simulink model "Inverter_circuit_redesign_from_NITW_Paper23_compatible"  (R2021a)
settings: Solver=ode23t  StartTime=0.0  StopTime=2  RelTol=1e-3
values from neighbouring files (symbols this model uses):
  B = 5    [FOC_parameters_Basil.m]    (also in parameters_FOC.m = 53)
  C_LCL = 100e-6    (= 0.0001)    [FOC_parameters_Basil.m]
  D = 0.25    [FOC_parameters_Basil.m]    (also in parameters_FOC.m)
  k = 1    [FOC_parameters_Basil.m]
  L_LCL = 500e-6    (= 0.0005)    [FOC_parameters_Basil.m]
  Ll = 0.0416    [FOC_parameters_Basil.m]
  Lm = 0.0416    [FOC_parameters_Basil.m]    (also in parameters_FOC.m = 0.4)
  Lp = 0.0684    [FOC_parameters_Basil.m]
  M = 4.775    [FOC_parameters_Basil.m]    (also in parameters_FOC.m)
  P = 2    [FOC_parameters_Basil.m]    (also in parameters_FOC.m = 4)
  Rl = 0.976    [FOC_parameters_Basil.m]
  Rp = 1.298    [FOC_parameters_Basil.m]
  Tp = 0.027    [FOC_parameters_Basil.m]    (also in parameters_FOC.m = 0.0465)
  VDC = 800    [FOC_parameters_Basil.m]
undefined symbols (not defined in the file or in its folder): L
libraries: spsSeriesRLCBranchLib x9, pid_lib x6, spsIGBTDiodeLib x6, eeTransforms x4, spsCurrentMeasurementLib x3, simulink_extras x1, spsDCVoltageSourceLib x1, simulink x1, spsThreePhaseVIMeasurementLib x1, spsdq0toabcLib x1, spspowerguiLib x1
(part 1 of 2)
settings Model: SimulationMode=accelerator  Creator=Basilisk  LastModifiedBy=Basilisk

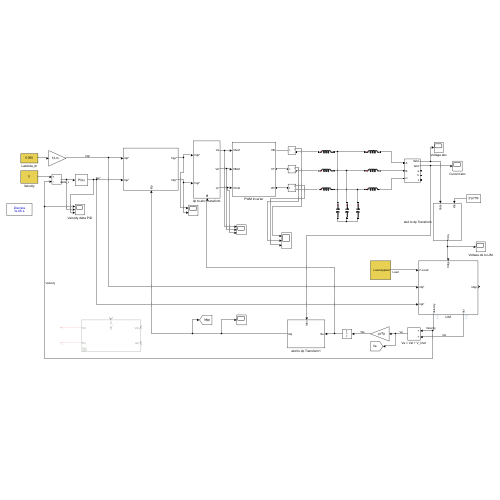
[thumbnail: Simulink's stored preview of the top-level diagram]
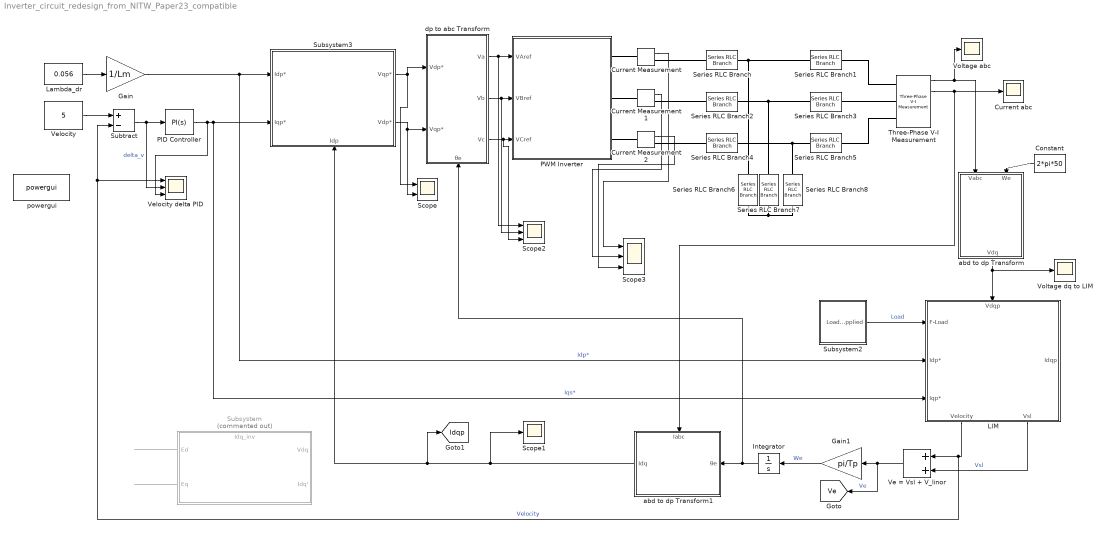
== system Inverter_circuit_redesign_from_NITW_Paper23_compatible ==
  Constant : Constant  Value=2*pi*50
  Current Measurement : spsCurrentMeasurementLib/Current Measurement  PhasorSimulation=off  OutputType=Complex  PSBequivalent=0
  Current Measurement1 : spsCurrentMeasurementLib/Current Measurement  PhasorSimulation=off  OutputType=Complex  PSBequivalent=0
  Current Measurement2 : spsCurrentMeasurementLib/Current Measurement  PhasorSimulation=off  OutputType=Complex  PSBequivalent=0
  Current abc : Scope
  Gain : Gain  Gain=1/Lm
  Gain1 : Gain  Gain=pi/Tp
  Integrator : Integrator
  LIM : Subsystem
      settings: PortSchema="{\"entries\":[{\"content\":{\"sides\":[{\"content\":{\"connectorIds\":[\"In1\",\"In2\",\"In3\"]},\"type\":\"ConnectorPlacement.EquallySpacedRectSide\",\"uuid\":\"f7446374-ee35-46fe-93ed-7921b6b2af41\"},{\"content\":{\"connectorIds\":[\"Out1\"],\"side\":\"RIGHT\"},\"type\":\"ConnectorPlacement.EquallySpacedRectSide\",\"uuid\":\"9c6022f9-7a1a-4d7e-a6a7-0d40c632aa44\"},{\"content\":{\"connectorIds\":[\"In4\"],\"side\":\"TOP\"},\"type\":\"ConnectorPlacement.EquallySpacedRectSide\",\"uuid\":\"61492046-b5c8-45e7-b8b1-17b26bfbb342\"},{\"content\":{\"connectorIds\":[\"Out2\",\"Out3\"],\"side\":\"BOTTOM\"},\"type\":\"ConnectorPlacement.EquallySpacedRectSide\",\"uuid\":\"5b9be1f1-04b7-4def-af6b-70d0d64eb3ec\"}]},\"type\":\"ConnectorPlacement.EquallySpacedConnector\",\"uuid\":\"408e196e-f76f-4ce9-bb6a-3d2dec3a79e2\"}],\"packageUris\":[\"http://schema.mathworks.com/mf0/Connector/R2020b\"],\"version\":\"1.0\"}"
  Lambda_dr : Constant  Value=0.056
  PID Controller : pid_lib/PID Controller  Controller=PI  Form=Parallel  TimeDomain=Continuous-time  UseExternalTs=off  SampleTime=-1  IntegratorMethod=Forward Euler  FilterMethod=Forward Euler  ControllerParametersSource=internal  P=10  I=5000  D=0  UseFilter=on  N=100  TunerSelectOption=Transfer Function Based (PID Tuner App)  InitialConditionSource=internal  InitialConditionForIntegrator=0  InitialConditionForFilter=0  DifferentiatorICPrevScaledInput=0  ExternalReset=none  TrackingMode=off  Kt=1  LimitOutput=off  SatLimitsSource=internal  UpperSaturationLimit=inf  LowerSaturationLimit=-inf  LinearizeAsGain=on  AntiWindupMode=none  Kb=1  POutMin=[]  POutMax=[]  IOutMin=[]  IOutMax=[]  DOutMin=[]  DOutMax=[]  NOutMin=[]  NOutMax=[]  SumOutMin=[]  SumOutMax=[]  SaturationOutMin=[]  SaturationOutMax=[]  PParamMin=[]  PParamMax=[]  IParamMin=[]  IParamMax=[]  DParamMin=[]  DParamMax=[]  NParamMin=[]  NParamMax=[]  KbParamMin=[]  KbParamMax=[]  KtParamMin=[]  KtParamMax=[]  KbOutMin=[]  KbOutMax=[]  KtOutMin=[]  KtOutMax=[]  IntegratorOutMin=[]  IntegratorOutMax=[]  FilterOutMin=[]  FilterOutMax=[]  SumI1OutMin=[]  SumI1OutMax=[]  SumI2OutMin=[]  SumI2OutMax=[]  SumI3OutMin=[]  SumI3OutMax=[]  SumI4OutMin=[]  SumI4OutMax=[]  SumDOutMin=[]  SumDOutMax=[]  DifferentiatorOutMin=[]  DifferentiatorOutMax=[]  FilterDiffOutCoefMin=[]  FilterDiffOutCoefMax=[]  ReciprocalOutMin=[]  ReciprocalOutMax=[]  SumDenOutMin=[]  SumDenOutMax=[]  SumNumOutMin=[]  SumNumOutMax=[]  DivideOutMin=[]  DivideOutMax=[]  UdiffTsProdOutMin=[]  UdiffTsProdOutMax=[]  NTsProdOutMin=[]  NTsProdOutMax=[]  UintegralTsProdOutMin=[]  UintegralTsProdOutMax=[]  UngainTsProdOutMin=[]  UngainTsProdOutMax=[]  IntegratorContinuousStateAttributes=''  IntegratorStateMustResolveToSignalObject=off  IntegratorRTWStateStorageClass=Auto  FilterContinuousStateAttributes=''  FilterStateMustResolveToSignalObject=off  FilterRTWStateStorageClass=Auto  ParallelPVariant=InternalParameters  IdealPVariant=Disabled  IVariant=InternalParameters  DVariant=Disabled  IntegratorVariant=Continuous  SatVariant=Disabled  AWVariant=Passthrough  PCopyVariant=Disabled  TRVariant=Disabled  FdbkBlocksVariant=Forward  IdealPFdbkVariant=Disabled  SatFdbkVariant=Disabled  DerivativeFilterVariant=Disabled  NVariant=Disabled  NCopyVariant=Disabled_SignalSpec  FilterICVariant=Disabled  IntegratorICVariant=InternalICs  ExternalResetVariant=Disabled  TRSumVariant=Passthrough  SumFdbkVariant=Disabled  SumVariant=Sum_PI  TsampFilterVariant=InternalTs  TsampNgainVariant=Passthrough  TsampIntegralVariant=Passthrough  ExternalSaturationOutDataTypeStr=Inherit: Same as second input
  PWM Inverter : Subsystem
  Scope : Scope  NumInputPorts=2
  Scope1 : Scope
  Scope2 : Scope  NumInputPorts=3
  Scope3 : Scope  NumInputPorts=3
  Series RLC Branch{,1..5} (6 alike) : spsSeriesRLCBranchLib/Series RLC Branch  LConnTagsString=__new0  RConnTagsString=__new0  BranchType=L  Resistance=1  Inductance=L_LCL  SetiL0=off  InitialCurrent=0  Capacitance=1e-6  Setx0=off  InitialVoltage=0  Measurements=None
  Series RLC Branch6 : spsSeriesRLCBranchLib/Series RLC Branch  LConnTagsString=__new0  RConnTagsString=__new0  BranchType=C  Resistance=1  Inductance=L  SetiL0=off  InitialCurrent=0  Capacitance=C_LCL  Setx0=off  InitialVoltage=0  Measurements=None
  Series RLC Branch7 : spsSeriesRLCBranchLib/Series RLC Branch  LConnTagsString=__new0  RConnTagsString=__new0  BranchType=C  Resistance=1  Inductance=L  SetiL0=off  InitialCurrent=0  Capacitance=C_LCL  Setx0=off  InitialVoltage=0  Measurements=None
  Series RLC Branch8 : spsSeriesRLCBranchLib/Series RLC Branch  LConnTagsString=__new0  RConnTagsString=__new0  BranchType=C  Resistance=1  Inductance=L  SetiL0=off  InitialCurrent=0  Capacitance=C_LCL  Setx0=off  InitialVoltage=0  Measurements=None
  Subsystem : Subsystem  Commented=on
      settings: PortSchema="{\"entries\":[{\"content\":{\"sides\":[{\"content\":{\"connectorIds\":[\"Out1\",\"Out2\"]},\"type\":\"ConnectorPlacement.EquallySpacedRectSide\",\"uuid\":\"49878900-a608-4033-9c06-f0f879ae24be\"},{\"content\":{\"connectorIds\":[\"In2\",\"In3\"],\"side\":\"RIGHT\"},\"type\":\"ConnectorPlacement.EquallySpacedRectSide\",\"uuid\":\"696fb92a-6e5e-4f05-bb0c-e09c99220dcc\"},{\"content\":{\"connectorIds\":[\"In1\"],\"side\":\"TOP\"},\"type\":\"ConnectorPlacement.EquallySpacedRectSide\",\"uuid\":\"dec37822-b677-40af-afbd-2d2c67f7ec3b\"}]},\"type\":\"ConnectorPlacement.EquallySpacedConnector\",\"uuid\":\"87482552-0ae1-4097-8c32-6cc01319ff44\"}],\"packageUris\":[\"http://schema.mathworks.com/mf0/Connector/R2020b\"],\"version\":\"1.0\"}"
  Subsystem2 : Subsystem
  Subsystem3 : Subsystem
      settings: PortSchema="{\"entries\":[{\"content\":{\"sides\":[{\"content\":{\"connectorIds\":[\"In1\",\"In2\"]},\"type\":\"ConnectorPlacement.EquallySpacedRectSide\",\"uuid\":\"297be966-0d57-4ba3-8372-2661d6cd0aff\"},{\"content\":{\"connectorIds\":[\"Out1\",\"Out2\"],\"side\":\"RIGHT\"},\"type\":\"ConnectorPlacement.EquallySpacedRectSide\",\"uuid\":\"6bb0515e-c942-4d41-9641-f6064e864ee1\"},{\"content\":{\"connectorIds\":[],\"side\":\"TOP\"},\"type\":\"ConnectorPlacement.EquallySpacedRectSide\",\"uuid\":\"b418268d-3115-4ff4-b82e-d56401585d58\"},{\"content\":{\"connectorIds\":[\"In3\"],\"side\":\"BOTTOM\"},\"type\":\"ConnectorPlacement.EquallySpacedRectSide\",\"uuid\":\"fdde8d49-e3fc-403e-acf2-e5bf672785bb\"}]},\"type\":\"ConnectorPlacement.EquallySpacedConnector\",\"uuid\":\"bea3ecdb-df2c-4728-adcd-4b82f3cb5d95\"}],\"packageUris\":[\"http://schema.mathworks.com/mf0/Connector/R2020b\"],\"version\":\"1.0\"}"
  Subtract : Sum  Inputs=+-
  Three-Phase V-I Measurement : spsThreePhaseVIMeasurementLib/Three-Phase V-I Measurement  VoltageMeasurement=phase-to-phase  SetLabelV=off  LabelV=Vabc  Vpu=off  VpuLL=off  CurrentMeasurement=yes  SetLabelI=off  LabelI=Iabc  Ipu=off  Pbase=100e6  Vbase=500e3  OutputType=Complex  PhasorSimulation=off  PSBequivalent=0
  Ve = Vsl + V_linor : Sum
  Velocity : Constant  Value=5
  Velocity delta PID : Scope  NumInputPorts=3
  Voltage abc : Scope
  Voltage dq to LIM : Scope
  abd to dp Transform : Subsystem
  abd to dp Transform1 : Subsystem
      settings: PortSchema="{\"entries\":[{\"content\":{\"sides\":[{\"content\":{\"connectorIds\":[\"Out1\"]},\"type\":\"ConnectorPlacement.EquallySpacedRectSide\",\"uuid\":\"0a5c08c4-5c41-497e-b18e-e04a9254d192\"},{\"content\":{\"connectorIds\":[\"In2\"],\"side\":\"RIGHT\"},\"type\":\"ConnectorPlacement.EquallySpacedRectSide\",\"uuid\":\"782de88f-5f2e-44b5-b7d6-55f2bd67aa91\"},{\"content\":{\"connectorIds\":[],\"side\":\"TOP\"},\"type\":\"ConnectorPlacement.EquallySpacedRectSide\",\"uuid\":\"cedc65d0-c52b-4972-ac1b-f9f495532484\"},{\"content\":{\"connectorIds\":[\"In1\"],\"side\":\"BOTTOM\"},\"type\":\"ConnectorPlacement.EquallySpacedRectSide\",\"uuid\":\"096e216c-1e33-4a9a-a102-8d40bb808988\"}]},\"type\":\"ConnectorPlacement.EquallySpacedConnector\",\"uuid\":\"2e2ddd2f-c989-4eb0-a4d7-2b4ecf545aeb\"}],\"packageUris\":[\"http://schema.mathworks.com/mf0/Connector/R2020b\"],\"version\":\"1.0\"}"
  dp to abc Transform : Subsystem
      settings: PortSchema="{\"entries\":[{\"content\":{\"sides\":[{\"content\":{\"connectorIds\":[\"In1\",\"In2\"]},\"type\":\"ConnectorPlacement.EquallySpacedRectSide\",\"uuid\":\"d8a782e4-9ec4-4209-9b4b-b1627326e2fd\"},{\"content\":{\"connectorIds\":[\"Out1\",\"Out2\",\"Out3\"],\"side\":\"RIGHT\"},\"type\":\"ConnectorPlacement.EquallySpacedRectSide\",\"uuid\":\"69fe3e47-1152-49e6-a7ef-958cf96a3504\"},{\"content\":{\"connectorIds\":[],\"side\":\"TOP\"},\"type\":\"ConnectorPlacement.EquallySpacedRectSide\",\"uuid\":\"f13122e8-6ec9-4b07-81b4-0ba679e15a5f\"},{\"content\":{\"connectorIds\":[\"In3\"],\"side\":\"BOTTOM\"},\"type\":\"ConnectorPlacement.EquallySpacedRectSide\",\"uuid\":\"3a3b978b-03f4-40da-8c91-f6bb64aea85e\"}]},\"type\":\"ConnectorPlacement.EquallySpacedConnector\",\"uuid\":\"570f73f2-39cb-4994-9999-9a17a3f46023\"}],\"packageUris\":[\"http://schema.mathworks.com/mf0/Connector/R2020b\"],\"version\":\"1.0\"}"
  powergui : spspowerguiLib/powergui  Priority=1  SimulationMode=Discrete  SampleTime=1e-6  frequency=60  Iterations=50  frequencyindice=0  Pbase=100e6  ErrMax=1e-4  UnitsV=kV  UnitsW=MW  buscounter=0  FunctionMessages=off  echomessages=off  EnableUseOfTLC=off  CurrentSourceSwitches=off  DisableSnubberDevices=off  DisableRonSwitches=off  DisableVfSwitches=off  DisplayEquations=off  AutomaticDiscreteSolvers=off  SolverType=Tustin/Backward Euler (TBE)  Interpol=off  ExternalGateDelay=off  methode=off  Ts=100  x0status=blocks  SPID=on  SwTol=0  HookPort=off  NonlinearTolerance=1e-4  nMaxIteration=100  ContinueOnMaxIteration=off  RestoreLinks=warning  ResistiveCurrentMeasurement=off  Frange=[0:2:500]  Ylog=off  Xlog=on  ShowGrid=off  save=off  variable=ZData  structure=0  ZoomFFT=off  StartTime=0.0  cycles=1  DisplayStyle=1  fundamental=60  FreqAxis=off  MaxFrequency=1000  frequencyindicesteady=1  RmsSteady=1  display=off
  tag scope: Idqp=global, Ve=global
  wires:
  abd to dp Transform/1(Vdq) -> Voltage dq to LIM/1, LIM/4(Vdqp)
  Constant/1 -> abd to dp Transform/1(We)
  Three-Phase V-I Measurement/1 -> Voltage abc/1, abd to dp Transform/2(Vabc)
  Subsystem/1(Ed) -> ?
  Subsystem/2(Eq) -> ?
  Velocity/1 -> Subtract/1
  Subsystem2/1(Load Applied) -> LIM/1(F-Load)  "Load"
  Integrator/1 -> abd to dp Transform1/2(θe), dp to abc Transform/3(θe)
  LIM/2(Velocity) -> Velocity delta PID/1, Subtract/2, Ve = Vsl + V_linor/1  "Velocity"
  LIM/3(Vsl) -> Ve = Vsl + V_linor/2  "Vsl"
  Subtract/1 -> PID Controller/1, Velocity delta PID/2  "delta_v"
  PID Controller/1 -> Velocity delta PID/3, LIM/3(Iqp*), Subsystem3/2(Iqp*)  "Iqs*"
  Lambda_dr/1 -> Gain/1
  Gain/1 -> LIM/2(Idp*), Subsystem3/1(Idp*)  "Idp*"
  Gain1/1 -> Integrator/1  "We"
  Ve = Vsl + V_linor/1 -> [Ve], Gain1/1  "Ve"
  Subsystem3/2(Vdp*) -> Scope/2, dp to abc Transform/2(Vqp*)
  Subsystem3/1(Vqp*) -> Scope/1, dp to abc Transform/1(Vdp*)
  dp to abc Transform/1(Va) -> Scope2/1, PWM Inverter/1(VAref)
  dp to abc Transform/2(Vb) -> Scope2/2, PWM Inverter/2(VBref)
  dp to abc Transform/3(Vc) -> Scope2/3, PWM Inverter/3(VCref)
  abd to dp Transform1/1(Idq) -> Scope1/1, [Idqp], Subsystem3/3(Idp)
  Three-Phase V-I Measurement/2 -> abd to dp Transform1/1(Iabc), Current abc/1
  Current Measurement/1 -> Scope3/1
  Current Measurement1/1 -> Scope3/2
  Current Measurement2/1 -> Scope3/3
  connections:
  Series RLC Branch/LConn1 -- Current Measurement/RConn1
  Series RLC Branch1/LConn1 -- Series RLC Branch6/LConn1 -- Series RLC Branch/RConn1
  Series RLC Branch2/LConn1 -- Current Measurement1/RConn1
  Series RLC Branch3/LConn1 -- Series RLC Branch2/RConn1 -- Series RLC Branch7/LConn1
  Series RLC Branch4/LConn1 -- Current Measurement2/RConn1
  Series RLC Branch5/LConn1 -- Series RLC Branch8/LConn1 -- Series RLC Branch4/RConn1
  Series RLC Branch6/RConn1 -- Series RLC Branch7/RConn1 -- Series RLC Branch8/RConn1
  Three-Phase V-I Measurement/LConn1 -- Series RLC Branch1/RConn1
  Three-Phase V-I Measurement/LConn2 -- Series RLC Branch3/RConn1
  Three-Phase V-I Measurement/LConn3 -- Series RLC Branch5/RConn1
  PWM Inverter/RConn1 -- Current Measurement/LConn1
  Current Measurement1/LConn1 -- PWM Inverter/RConn2
  PWM Inverter/RConn3 -- Current Measurement2/LConn1

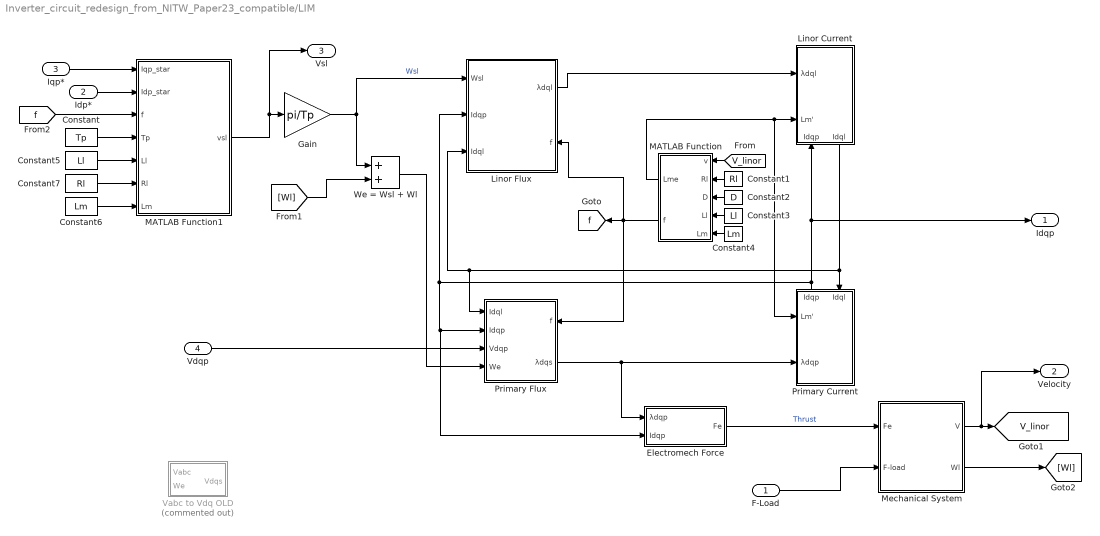
== system Inverter_circuit_redesign_from_NITW_Paper23_compatible/LIM ==
  F-Load : Inport
  Idp* : Inport  Port=2
  Iqp* : Inport  Port=3
  Vdqp : Inport  Port=4
  Constant : Constant  Value=Tp
  Constant1 : Constant  Value=Rl
  Constant2 : Constant  Value=D
  Constant3 : Constant  Value=Ll
  Constant4 : Constant  Value=Lm
  Constant5 : Constant  Value=Ll
  Constant6 : Constant  Value=Lm
  Constant7 : Constant  Value=Rl
  Electromech Force : Subsystem
  Gain : Gain  Gain=pi/Tp
  Linor Current : Subsystem
      settings: PortSchema="{\"entries\":[{\"content\":{\"sides\":[{\"content\":{\"connectorIds\":[\"In1\",\"In2\"]},\"type\":\"ConnectorPlacement.EquallySpacedRectSide\",\"uuid\":\"40d9865c-3cfa-44c1-93eb-682b1c6628f3\"},{\"content\":{\"connectorIds\":[],\"side\":\"RIGHT\"},\"type\":\"ConnectorPlacement.EquallySpacedRectSide\",\"uuid\":\"35710d59-e170-4e3b-9d71-9b17ce19d5d9\"},{\"content\":{\"connectorIds\":[],\"side\":\"TOP\"},\"type\":\"ConnectorPlacement.EquallySpacedRectSide\",\"uuid\":\"24aa0d2b-de57-4aff-b066-c7bd8ef57638\"},{\"content\":{\"connectorIds\":[\"In3\",\"Out1\"],\"side\":\"BOTTOM\"},\"type\":\"ConnectorPlacement.EquallySpacedRectSide\",\"uuid\":\"ba21e6b6-d163-44f4-8ede-2a2a18cab7d2\"}]},\"type\":\"ConnectorPlacement.EquallySpacedConnector\",\"uuid\":\"7a74cd09-26a1-4394-b388-2a31d7083798\"}],\"packageUris\":[\"http://schema.mathworks.com/mf0/Connector/R2020b\"],\"version\":\"1.0\"}"
  Linor Flux : Subsystem
      settings: PortSchema="{\"entries\":[{\"content\":{\"sides\":[{\"content\":{\"connectorIds\":[\"In1\",\"In2\",\"In3\"]},\"type\":\"ConnectorPlacement.EquallySpacedRectSide\",\"uuid\":\"b9a9f404-9b3b-4182-a50e-1bf7cef191e8\"},{\"content\":{\"connectorIds\":[\"Out1\",\"In4\"],\"side\":\"RIGHT\"},\"type\":\"ConnectorPlacement.EquallySpacedRectSide\",\"uuid\":\"68159d79-7975-4fd0-98a3-7e35432781a2\"},{\"content\":{\"connectorIds\":[],\"side\":\"TOP\"},\"type\":\"ConnectorPlacement.EquallySpacedRectSide\",\"uuid\":\"0c4dbb5d-b4d4-4876-b829-49090bd6eeb8\"},{\"content\":{\"connectorIds\":[],\"side\":\"HIDDEN\"},\"type\":\"ConnectorPlacement.EquallySpacedRectSide\",\"uuid\":\"f2a65973-682a-4dd6-b429-3fa72198cae4\"}]},\"type\":\"ConnectorPlacement.EquallySpacedConnector\",\"uuid\":\"744eb17f-cf6a-4151-90db-78263b57d619\"}],\"packageUris\":[\"http://schema.mathworks.com/mf0/Connector/R2020b\"],\"version\":\"1.0\"}"
  MATLAB Function : MATLAB Function  TreatAsAtomicUnit=on
  MATLAB Function1 : MATLAB Function  TreatAsAtomicUnit=on
  Mechanical System : Subsystem
  Primary Current : Subsystem
      settings: PortSchema="{\"entries\":[{\"content\":{\"sides\":[{\"content\":{\"connectorIds\":[\"In1\",\"In2\"]},\"type\":\"ConnectorPlacement.EquallySpacedRectSide\",\"uuid\":\"40d9865c-3cfa-44c1-93eb-682b1c6628f3\"},{\"content\":{\"connectorIds\":[],\"side\":\"RIGHT\"},\"type\":\"ConnectorPlacement.EquallySpacedRectSide\",\"uuid\":\"35710d59-e170-4e3b-9d71-9b17ce19d5d9\"},{\"content\":{\"connectorIds\":[\"Out1\",\"In3\"],\"side\":\"TOP\"},\"type\":\"ConnectorPlacement.EquallySpacedRectSide\",\"uuid\":\"24aa0d2b-de57-4aff-b066-c7bd8ef57638\"}]},\"type\":\"ConnectorPlacement.EquallySpacedConnector\",\"uuid\":\"7a74cd09-26a1-4394-b388-2a31d7083798\"}],\"packageUris\":[\"http://schema.mathworks.com/mf0/Connector/R2020b\"],\"version\":\"1.0\"}"
  Primary Flux : Subsystem
      settings: PortSchema="{\"entries\":[{\"content\":{\"sides\":[{\"content\":{\"connectorIds\":[\"In1\",\"In2\",\"In3\",\"In4\"]},\"type\":\"ConnectorPlacement.EquallySpacedRectSide\",\"uuid\":\"a4b29cca-9cb0-4324-9244-2049ffc93668\"},{\"content\":{\"connectorIds\":[\"In5\",\"Out1\"],\"side\":\"RIGHT\"},\"type\":\"ConnectorPlacement.EquallySpacedRectSide\",\"uuid\":\"b20ff3ac-d40e-4f59-bb91-f6f2c0c6ca63\"},{\"content\":{\"connectorIds\":[],\"side\":\"TOP\"},\"type\":\"ConnectorPlacement.EquallySpacedRectSide\",\"uuid\":\"55342d43-b8f9-4aa9-846c-26670e92f4ca\"},{\"content\":{\"connectorIds\":[],\"side\":\"HIDDEN\"},\"type\":\"ConnectorPlacement.EquallySpacedRectSide\",\"uuid\":\"5fed22a0-a45a-430c-a997-0be85a9315bb\"}]},\"type\":\"ConnectorPlacement.EquallySpacedConnector\",\"uuid\":\"78d5652d-2b6b-4c50-974b-d09ad892483f\"}],\"packageUris\":[\"http://schema.mathworks.com/mf0/Connector/R2020b\"],\"version\":\"1.0\"}"
  "Vabc to Vdq OLD " : Subsystem  Commented=on
  We = Wsl + Wl : Sum
  Idqp : Outport
  Velocity : Outport  Port=2
  Vsl : Outport  Port=3
  tag scope: V_linor=global, f=global
  wires:
  Primary Flux/1(λdqs) -> Electromech Force/1(λdqp), Primary Current/2(λdqp)
  Vdqp/1 -> Primary Flux/3(Vdqp)
  [V_linor] -> MATLAB Function/1(v)
  Constant3/1 -> MATLAB Function/4(Ll)
  Constant2/1 -> MATLAB Function/3(D)
  Constant4/1 -> MATLAB Function/5(Lm)
  Constant1/1 -> MATLAB Function/2(Rl)
  MATLAB Function/2(f) -> Primary Flux/5(f), [f], Linor Flux/4(f)
  Linor Flux/1(λdql) -> Linor Current/1(λdql)
  MATLAB Function/1(Lme) -> Primary Current/1(Lm'), Linor Current/2(Lm')
  Linor Current/1(Idql) -> Primary Flux/1(Idql), Linor Flux/3(Idql), Primary Current/3(Idql)
  Primary Current/1(Idqp) -> Idqp/1, Linor Current/3(Idqp), Primary Flux/2(Idqp), Electromech Force/2(Idqp), Linor Flux/2(Idqp)
  Electromech Force/1(Fe) -> Mechanical System/1(Fe)  "Thrust"
  F-Load/1 -> Mechanical System/2(F-load)
  Mechanical System/1(V) -> Velocity/1, [V_linor]
  Mechanical System/2(Wl) -> [Wl]
  We = Wsl + Wl/1 -> Primary Flux/4(We)
  [Wl] -> We = Wsl + Wl/2
  Gain/1 -> Linor Flux/1(Wsl), We = Wsl + Wl/1  "Wsl"
  MATLAB Function1/1(vsl) -> Vsl/1, Gain/1
  Iqp*/1 -> MATLAB Function1/1(Iqp_star)
  Idp*/1 -> MATLAB Function1/2(Idp_star)
  [f] -> MATLAB Function1/3(f)
  Constant7/1 -> MATLAB Function1/6(Rl)
  Constant6/1 -> MATLAB Function1/7(Lm)
  Constant5/1 -> MATLAB Function1/5(Ll)
  Constant/1 -> MATLAB Function1/4(Tp)

== system Inverter_circuit_redesign_from_NITW_Paper23_compatible/PWM Inverter ==
  VAref : Inport
  VBref : Inport  Port=2
  VCref : Inport  Port=3
  "DC Voltage Source " : spsDCVoltageSourceLib/DC Voltage Source  Amplitude=VDC  Measurements=None
  Inverter : Subsystem
  PMW : Subsystem
      settings: PortSchema="{\"entries\":[{\"content\":{\"sides\":[{\"content\":{\"connectorIds\":[\"Out1\",\"Out2\",\"Out3\"]},\"type\":\"ConnectorPlacement.EquallySpacedRectSide\",\"uuid\":\"fa5038a1-afc0-4dd0-b72d-009c2412aee1\"},{\"content\":{\"connectorIds\":[\"In1\",\"In2\",\"In3\"],\"side\":\"RIGHT\"},\"type\":\"ConnectorPlacement.EquallySpacedRectSide\",\"uuid\":\"b873ef02-5cf0-4d47-90da-8e56690c29fa\"},{\"content\":{\"connectorIds\":[],\"side\":\"TOP\"},\"type\":\"ConnectorPlacement.EquallySpacedRectSide\",\"uuid\":\"2e4c823b-e436-4a61-b8d9-aeb5834b7046\"}]},\"type\":\"ConnectorPlacement.EquallySpacedConnector\",\"uuid\":\"f2dc5969-6286-4fa7-a133-dd46c0b75d70\"}],\"packageUris\":[\"http://schema.mathworks.com/mf0/Connector/R2020b\"],\"version\":\"1.0\"}"
  VB : PMIOPort  Side=Right
  VY : PMIOPort  Port=2  Side=Right
  VR : PMIOPort  Port=3  Side=Right
  wires:
  PMW/1(PWM3) -> Inverter/3(PWM3)
  PMW/2(PWM2) -> Inverter/2(PWM2)
  PMW/3(PWM1) -> Inverter/1(PWM1)
  VAref/1 -> PMW/1(VAref)
  VCref/1 -> PMW/3(VCref)
  VBref/1 -> PMW/2(VBref)
  connections:
  "DC Voltage Source "/LConn1 -- Inverter/LConn2
  "DC Voltage Source "/RConn1 -- Inverter/LConn1
  Inverter/RConn3 -- VR/RConn1
  VY/RConn1 -- Inverter/RConn2
  Inverter/RConn1 -- VB/RConn1

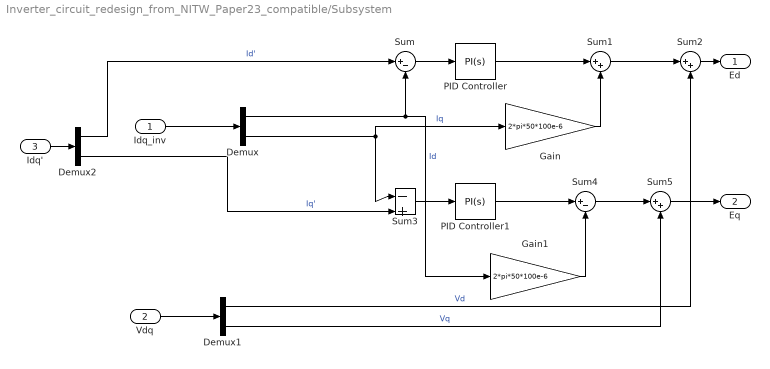
== system Inverter_circuit_redesign_from_NITW_Paper23_compatible/Subsystem ==
  Idq_inv : Inport
  Vdq : Inport  Port=2
  Idq' : Inport  Port=3
  Demux : Demux  Outputs=2
  Demux1 : Demux  Outputs=2
  Demux2 : Demux  Outputs=2
  Gain : Gain  Gain=2*pi*50*100e-6
  Gain1 : Gain  Gain=2*pi*50*100e-6
  PID Controller : pid_lib/PID Controller  Controller=PI  Form=Parallel  TimeDomain=Continuous-time  UseExternalTs=off  SampleTime=-1  IntegratorMethod=Forward Euler  FilterMethod=Forward Euler  ControllerParametersSource=internal  P=5  I=5000  D=0  UseFilter=on  N=100  TunerSelectOption=Transfer Function Based (PID Tuner App)  InitialConditionSource=internal  InitialConditionForIntegrator=0  InitialConditionForFilter=0  DifferentiatorICPrevScaledInput=0  ExternalReset=none  TrackingMode=off  Kt=1  LimitOutput=off  SatLimitsSource=internal  UpperSaturationLimit=inf  LowerSaturationLimit=-inf  LinearizeAsGain=on  AntiWindupMode=none  Kb=1  POutMin=[]  POutMax=[]  IOutMin=[]  IOutMax=[]  DOutMin=[]  DOutMax=[]  NOutMin=[]  NOutMax=[]  SumOutMin=[]  SumOutMax=[]  SaturationOutMin=[]  SaturationOutMax=[]  PParamMin=[]  PParamMax=[]  IParamMin=[]  IParamMax=[]  DParamMin=[]  DParamMax=[]  NParamMin=[]  NParamMax=[]  KbParamMin=[]  KbParamMax=[]  KtParamMin=[]  KtParamMax=[]  KbOutMin=[]  KbOutMax=[]  KtOutMin=[]  KtOutMax=[]  IntegratorOutMin=[]  IntegratorOutMax=[]  FilterOutMin=[]  FilterOutMax=[]  SumI1OutMin=[]  SumI1OutMax=[]  SumI2OutMin=[]  SumI2OutMax=[]  SumI3OutMin=[]  SumI3OutMax=[]  SumI4OutMin=[]  SumI4OutMax=[]  SumDOutMin=[]  SumDOutMax=[]  DifferentiatorOutMin=[]  DifferentiatorOutMax=[]  FilterDiffOutCoefMin=[]  FilterDiffOutCoefMax=[]  ReciprocalOutMin=[]  ReciprocalOutMax=[]  SumDenOutMin=[]  SumDenOutMax=[]  SumNumOutMin=[]  SumNumOutMax=[]  DivideOutMin=[]  DivideOutMax=[]  UdiffTsProdOutMin=[]  UdiffTsProdOutMax=[]  NTsProdOutMin=[]  NTsProdOutMax=[]  UintegralTsProdOutMin=[]  UintegralTsProdOutMax=[]  UngainTsProdOutMin=[]  UngainTsProdOutMax=[]  IntegratorContinuousStateAttributes=''  IntegratorStateMustResolveToSignalObject=off  IntegratorRTWStateStorageClass=Auto  FilterContinuousStateAttributes=''  FilterStateMustResolveToSignalObject=off  FilterRTWStateStorageClass=Auto  ParallelPVariant=InternalParameters  IdealPVariant=Disabled  IVariant=InternalParameters  DVariant=Disabled  IntegratorVariant=Continuous  SatVariant=Disabled  AWVariant=Passthrough  PCopyVariant=Disabled  TRVariant=Disabled  FdbkBlocksVariant=Forward  IdealPFdbkVariant=Disabled  SatFdbkVariant=Disabled  DerivativeFilterVariant=Disabled  NVariant=Disabled  NCopyVariant=Disabled_SignalSpec  FilterICVariant=Disabled  IntegratorICVariant=InternalICs  ExternalResetVariant=Disabled  TRSumVariant=Passthrough  SumFdbkVariant=Disabled  SumVariant=Sum_PI  TsampFilterVariant=InternalTs  TsampNgainVariant=Passthrough  TsampIntegralVariant=Passthrough  ExternalSaturationOutDataTypeStr=Inherit: Same as second input
  PID Controller1 : pid_lib/PID Controller  Controller=PI  Form=Parallel  TimeDomain=Continuous-time  UseExternalTs=off  SampleTime=-1  IntegratorMethod=Forward Euler  FilterMethod=Forward Euler  ControllerParametersSource=internal  P=5  I=5000  D=0  UseFilter=on  N=100  TunerSelectOption=Transfer Function Based (PID Tuner App)  InitialConditionSource=internal  InitialConditionForIntegrator=0  InitialConditionForFilter=0  DifferentiatorICPrevScaledInput=0  ExternalReset=none  TrackingMode=off  Kt=1  LimitOutput=off  SatLimitsSource=internal  UpperSaturationLimit=inf  LowerSaturationLimit=-inf  LinearizeAsGain=on  AntiWindupMode=none  Kb=1  POutMin=[]  POutMax=[]  IOutMin=[]  IOutMax=[]  DOutMin=[]  DOutMax=[]  NOutMin=[]  NOutMax=[]  SumOutMin=[]  SumOutMax=[]  SaturationOutMin=[]  SaturationOutMax=[]  PParamMin=[]  PParamMax=[]  IParamMin=[]  IParamMax=[]  DParamMin=[]  DParamMax=[]  NParamMin=[]  NParamMax=[]  KbParamMin=[]  KbParamMax=[]  KtParamMin=[]  KtParamMax=[]  KbOutMin=[]  KbOutMax=[]  KtOutMin=[]  KtOutMax=[]  IntegratorOutMin=[]  IntegratorOutMax=[]  FilterOutMin=[]  FilterOutMax=[]  SumI1OutMin=[]  SumI1OutMax=[]  SumI2OutMin=[]  SumI2OutMax=[]  SumI3OutMin=[]  SumI3OutMax=[]  SumI4OutMin=[]  SumI4OutMax=[]  SumDOutMin=[]  SumDOutMax=[]  DifferentiatorOutMin=[]  DifferentiatorOutMax=[]  FilterDiffOutCoefMin=[]  FilterDiffOutCoefMax=[]  ReciprocalOutMin=[]  ReciprocalOutMax=[]  SumDenOutMin=[]  SumDenOutMax=[]  SumNumOutMin=[]  SumNumOutMax=[]  DivideOutMin=[]  DivideOutMax=[]  UdiffTsProdOutMin=[]  UdiffTsProdOutMax=[]  NTsProdOutMin=[]  NTsProdOutMax=[]  UintegralTsProdOutMin=[]  UintegralTsProdOutMax=[]  UngainTsProdOutMin=[]  UngainTsProdOutMax=[]  IntegratorContinuousStateAttributes=''  IntegratorStateMustResolveToSignalObject=off  IntegratorRTWStateStorageClass=Auto  FilterContinuousStateAttributes=''  FilterStateMustResolveToSignalObject=off  FilterRTWStateStorageClass=Auto  ParallelPVariant=InternalParameters  IdealPVariant=Disabled  IVariant=InternalParameters  DVariant=Disabled  IntegratorVariant=Continuous  SatVariant=Disabled  AWVariant=Passthrough  PCopyVariant=Disabled  TRVariant=Disabled  FdbkBlocksVariant=Forward  IdealPFdbkVariant=Disabled  SatFdbkVariant=Disabled  DerivativeFilterVariant=Disabled  NVariant=Disabled  NCopyVariant=Disabled_SignalSpec  FilterICVariant=Disabled  IntegratorICVariant=InternalICs  ExternalResetVariant=Disabled  TRSumVariant=Passthrough  SumFdbkVariant=Disabled  SumVariant=Sum_PI  TsampFilterVariant=InternalTs  TsampNgainVariant=Passthrough  TsampIntegralVariant=Passthrough  ExternalSaturationOutDataTypeStr=Inherit: Same as second input
  Sum : Sum  Inputs=|+-
  Sum1 : Sum  Inputs=|++
  Sum2 : Sum  Inputs=|++
  Sum3 : Sum  Inputs=|-+
  Sum4 : Sum  Inputs=|+-
  Sum5 : Sum  Inputs=|++
  Ed : Outport
  Eq : Outport  Port=2
  wires:
  Sum3/1 -> PID Controller1/1
  Gain/1 -> Sum1/2
  PID Controller/1 -> Sum1/1
  Sum1/1 -> Sum2/1
  PID Controller1/1 -> Sum4/1
  Sum/1 -> PID Controller/1
  Gain1/1 -> Sum4/2
  Sum4/1 -> Sum5/1
  Demux/1 -> Gain1/1, Sum/2  "Id"
  Demux/2 -> Sum3/1, Gain/1  "Iq"
  Sum2/1 -> Ed/1
  Sum5/1 -> Eq/1
  Idq_inv/1 -> Demux/1
  Demux2/2 -> Sum3/2  "Iq'"
  Vdq/1 -> Demux1/1
  Demux1/1 -> Sum2/2  "Vd"
  Demux1/2 -> Sum5/2  "Vq"
  Idq'/1 -> Demux2/1
  Demux2/1 -> Sum/1  "Id'"

== system Inverter_circuit_redesign_from_NITW_Paper23_compatible/Subsystem2 ==
  note: Load Applied
  Add1 : Sum  Inputs=++++
  Constant3 : Constant  Value=5
  Manual Switch1 : ManualSwitch
  Step1 : Step  Time=0.5  After=40  SampleTime=0
  Step5 : Step  Time=0.9  After=100  SampleTime=0
  Step6 : Step  Time=2  After=200  SampleTime=0
  Step7 : Step  Time=1.5  After=600  SampleTime=0
  Load Applied : Outport
  wires:
  Step6/1 -> Add1/4
  Step7/1 -> Add1/3
  Step5/1 -> Add1/2
  Step1/1 -> Add1/1
  Add1/1 -> Manual Switch1/2
  Constant3/1 -> Manual Switch1/1
  Manual Switch1/1 -> Load Applied/1  "Load Applied"

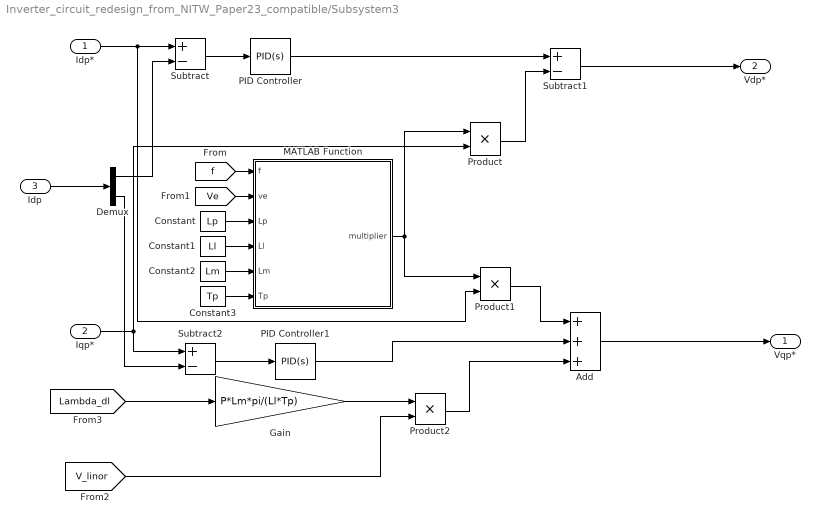
== system Inverter_circuit_redesign_from_NITW_Paper23_compatible/Subsystem3 ==
  Idp* : Inport
  Iqp* : Inport  Port=2
  Idp : Inport  Port=3
  Add : Sum  Inputs=+++
  Constant : Constant  Value=Lp
  Constant1 : Constant  Value=Ll
  Constant2 : Constant  Value=Lm
  Constant3 : Constant  Value=Tp
  Demux : Demux  Outputs=2
  Gain : Gain  Gain=P*Lm*pi/(Ll*Tp)
  MATLAB Function : MATLAB Function  TreatAsAtomicUnit=on
  PID Controller : pid_lib/PID Controller  Controller=PID  Form=Parallel  TimeDomain=Continuous-time  UseExternalTs=off  SampleTime=-1  IntegratorMethod=Forward Euler  FilterMethod=Forward Euler  ControllerParametersSource=internal  P=1  I=50  D=5  UseFilter=on  N=100  TunerSelectOption=Transfer Function Based (PID Tuner App)  InitialConditionSource=internal  InitialConditionForIntegrator=0  InitialConditionForFilter=0  DifferentiatorICPrevScaledInput=0  ExternalReset=none  TrackingMode=off  Kt=1  LimitOutput=off  SatLimitsSource=internal  UpperSaturationLimit=inf  LowerSaturationLimit=-inf  LinearizeAsGain=on  AntiWindupMode=none  Kb=1  POutMin=[]  POutMax=[]  IOutMin=[]  IOutMax=[]  DOutMin=[]  DOutMax=[]  NOutMin=[]  NOutMax=[]  SumOutMin=[]  SumOutMax=[]  SaturationOutMin=[]  SaturationOutMax=[]  PParamMin=[]  PParamMax=[]  IParamMin=[]  IParamMax=[]  DParamMin=[]  DParamMax=[]  NParamMin=[]  NParamMax=[]  KbParamMin=[]  KbParamMax=[]  KtParamMin=[]  KtParamMax=[]  KbOutMin=[]  KbOutMax=[]  KtOutMin=[]  KtOutMax=[]  IntegratorOutMin=[]  IntegratorOutMax=[]  FilterOutMin=[]  FilterOutMax=[]  SumI1OutMin=[]  SumI1OutMax=[]  SumI2OutMin=[]  SumI2OutMax=[]  SumI3OutMin=[]  SumI3OutMax=[]  SumI4OutMin=[]  SumI4OutMax=[]  SumDOutMin=[]  SumDOutMax=[]  DifferentiatorOutMin=[]  DifferentiatorOutMax=[]  FilterDiffOutCoefMin=[]  FilterDiffOutCoefMax=[]  ReciprocalOutMin=[]  ReciprocalOutMax=[]  SumDenOutMin=[]  SumDenOutMax=[]  SumNumOutMin=[]  SumNumOutMax=[]  DivideOutMin=[]  DivideOutMax=[]  UdiffTsProdOutMin=[]  UdiffTsProdOutMax=[]  NTsProdOutMin=[]  NTsProdOutMax=[]  UintegralTsProdOutMin=[]  UintegralTsProdOutMax=[]  UngainTsProdOutMin=[]  UngainTsProdOutMax=[]  IntegratorContinuousStateAttributes=''  IntegratorStateMustResolveToSignalObject=off  IntegratorRTWStateStorageClass=Auto  FilterContinuousStateAttributes=''  FilterStateMustResolveToSignalObject=off  FilterRTWStateStorageClass=Auto  ParallelPVariant=InternalParameters  IdealPVariant=Disabled  IVariant=InternalParameters  DVariant=InternalParameters  IntegratorVariant=Continuous  SatVariant=Disabled  AWVariant=Passthrough  PCopyVariant=Disabled  TRVariant=Disabled  FdbkBlocksVariant=Forward  IdealPFdbkVariant=Disabled  SatFdbkVariant=Disabled  DerivativeFilterVariant=ContFilter  NVariant=InternalParameters  NCopyVariant=Disabled  FilterICVariant=InternalICsFilter  IntegratorICVariant=InternalICs  ExternalResetVariant=Disabled  TRSumVariant=Passthrough  SumFdbkVariant=Disabled  SumVariant=Sum_PID  TsampFilterVariant=InternalTs  TsampNgainVariant=Passthrough  TsampIntegralVariant=Passthrough  ExternalSaturationOutDataTypeStr=Inherit: Same as second input
  PID Controller1 : pid_lib/PID Controller  Controller=PID  Form=Parallel  TimeDomain=Continuous-time  UseExternalTs=off  SampleTime=-1  IntegratorMethod=Forward Euler  FilterMethod=Forward Euler  ControllerParametersSource=internal  P=1  I=50  D=5  UseFilter=on  N=100  TunerSelectOption=Transfer Function Based (PID Tuner App)  InitialConditionSource=internal  InitialConditionForIntegrator=0  InitialConditionForFilter=0  DifferentiatorICPrevScaledInput=0  ExternalReset=none  TrackingMode=off  Kt=1  LimitOutput=off  SatLimitsSource=internal  UpperSaturationLimit=inf  LowerSaturationLimit=-inf  LinearizeAsGain=on  AntiWindupMode=none  Kb=1  POutMin=[]  POutMax=[]  IOutMin=[]  IOutMax=[]  DOutMin=[]  DOutMax=[]  NOutMin=[]  NOutMax=[]  SumOutMin=[]  SumOutMax=[]  SaturationOutMin=[]  SaturationOutMax=[]  PParamMin=[]  PParamMax=[]  IParamMin=[]  IParamMax=[]  DParamMin=[]  DParamMax=[]  NParamMin=[]  NParamMax=[]  KbParamMin=[]  KbParamMax=[]  KtParamMin=[]  KtParamMax=[]  KbOutMin=[]  KbOutMax=[]  KtOutMin=[]  KtOutMax=[]  IntegratorOutMin=[]  IntegratorOutMax=[]  FilterOutMin=[]  FilterOutMax=[]  SumI1OutMin=[]  SumI1OutMax=[]  SumI2OutMin=[]  SumI2OutMax=[]  SumI3OutMin=[]  SumI3OutMax=[]  SumI4OutMin=[]  SumI4OutMax=[]  SumDOutMin=[]  SumDOutMax=[]  DifferentiatorOutMin=[]  DifferentiatorOutMax=[]  FilterDiffOutCoefMin=[]  FilterDiffOutCoefMax=[]  ReciprocalOutMin=[]  ReciprocalOutMax=[]  SumDenOutMin=[]  SumDenOutMax=[]  SumNumOutMin=[]  SumNumOutMax=[]  DivideOutMin=[]  DivideOutMax=[]  UdiffTsProdOutMin=[]  UdiffTsProdOutMax=[]  NTsProdOutMin=[]  NTsProdOutMax=[]  UintegralTsProdOutMin=[]  UintegralTsProdOutMax=[]  UngainTsProdOutMin=[]  UngainTsProdOutMax=[]  IntegratorContinuousStateAttributes=''  IntegratorStateMustResolveToSignalObject=off  IntegratorRTWStateStorageClass=Auto  FilterContinuousStateAttributes=''  FilterStateMustResolveToSignalObject=off  FilterRTWStateStorageClass=Auto  ParallelPVariant=InternalParameters  IdealPVariant=Disabled  IVariant=InternalParameters  DVariant=InternalParameters  IntegratorVariant=Continuous  SatVariant=Disabled  AWVariant=Passthrough  PCopyVariant=Disabled  TRVariant=Disabled  FdbkBlocksVariant=Forward  IdealPFdbkVariant=Disabled  SatFdbkVariant=Disabled  DerivativeFilterVariant=ContFilter  NVariant=InternalParameters  NCopyVariant=Disabled  FilterICVariant=InternalICsFilter  IntegratorICVariant=InternalICs  ExternalResetVariant=Disabled  TRSumVariant=Passthrough  SumFdbkVariant=Disabled  SumVariant=Sum_PID  TsampFilterVariant=InternalTs  TsampNgainVariant=Passthrough  TsampIntegralVariant=Passthrough  ExternalSaturationOutDataTypeStr=Inherit: Same as second input
  Product : Product
  Product1 : Product
  Product2 : Product
  Subtract : Sum  Inputs=+-
  Subtract1 : Sum  Inputs=+-
  Subtract2 : Sum  Inputs=+-
  Vqp* : Outport
  Vdp* : Outport  Port=2
  wires:
  Idp/1 -> Demux/1
  Idp*/1 -> Product1/2, Subtract/1
  Demux/1 -> Subtract/2
  Subtract/1 -> PID Controller/1
  [f] -> MATLAB Function/1(f)
  PID Controller/1 -> Subtract1/1
  MATLAB Function/1(multiplier) -> Product/1, Product1/1
  [Ve] -> MATLAB Function/2(ve)
  Product/1 -> Subtract1/2
  Subtract1/1 -> Vdp*/1
  Subtract2/1 -> PID Controller1/1
  Iqp*/1 -> Product/2, Subtract2/1
  Demux/2 -> Subtract2/2
  PID Controller1/1 -> Add/2
  Add/1 -> Vqp*/1
  Product1/1 -> Add/1
  Product2/1 -> Add/3
  [V_linor] -> Product2/2
  [Lambda_dl] -> Gain/1
  Gain/1 -> Product2/1
  Constant1/1 -> MATLAB Function/4(Ll)
  Constant/1 -> MATLAB Function/3(Lp)
  Constant2/1 -> MATLAB Function/5(Lm)
  Constant3/1 -> MATLAB Function/6(Tp)

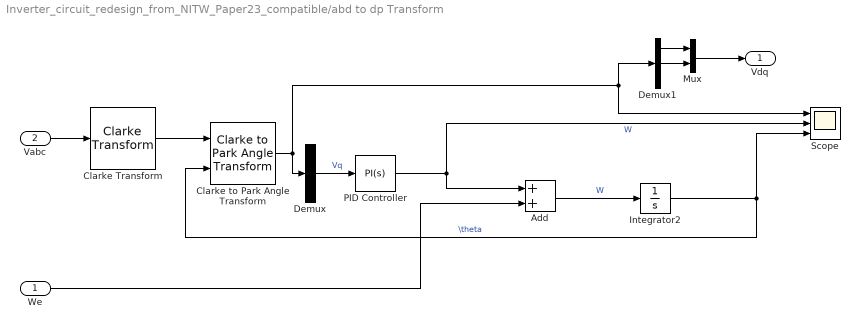
== system Inverter_circuit_redesign_from_NITW_Paper23_compatible/abd to dp Transform ==
  We : Inport
  Vabc : Inport  Port=2
  Add : Sum
  Clarke Transform : eeTransforms/Clarke Transform  PowerInvariant=off
      settings: SourceProductBaseCode=PS
  Clarke to Park Angle Transform : eeTransforms/Clarke to Park Angle Transform  AxisAlignment=Q-axis
      settings: SourceProductBaseCode=PS
  Demux : Demux  Outputs=3
  Demux1 : Demux  Outputs=3
  Integrator2 : Integrator
  Mux : Mux  Inputs=2
  PID Controller : pid_lib/PID Controller  Controller=PI  Form=Parallel  TimeDomain=Continuous-time  UseExternalTs=off  SampleTime=-1  IntegratorMethod=Forward Euler  FilterMethod=Forward Euler  ControllerParametersSource=internal  P=10  I=50000  D=0  UseFilter=on  N=100  TunerSelectOption=Transfer Function Based (PID Tuner App)  InitialConditionSource=internal  InitialConditionForIntegrator=0  InitialConditionForFilter=0  DifferentiatorICPrevScaledInput=0  ExternalReset=none  TrackingMode=off  Kt=1  LimitOutput=off  SatLimitsSource=internal  UpperSaturationLimit=inf  LowerSaturationLimit=-inf  LinearizeAsGain=on  AntiWindupMode=none  Kb=1  POutMin=[]  POutMax=[]  IOutMin=[]  IOutMax=[]  DOutMin=[]  DOutMax=[]  NOutMin=[]  NOutMax=[]  SumOutMin=[]  SumOutMax=[]  SaturationOutMin=[]  SaturationOutMax=[]  PParamMin=[]  PParamMax=[]  IParamMin=[]  IParamMax=[]  DParamMin=[]  DParamMax=[]  NParamMin=[]  NParamMax=[]  KbParamMin=[]  KbParamMax=[]  KtParamMin=[]  KtParamMax=[]  KbOutMin=[]  KbOutMax=[]  KtOutMin=[]  KtOutMax=[]  IntegratorOutMin=[]  IntegratorOutMax=[]  FilterOutMin=[]  FilterOutMax=[]  SumI1OutMin=[]  SumI1OutMax=[]  SumI2OutMin=[]  SumI2OutMax=[]  SumI3OutMin=[]  SumI3OutMax=[]  SumI4OutMin=[]  SumI4OutMax=[]  SumDOutMin=[]  SumDOutMax=[]  DifferentiatorOutMin=[]  DifferentiatorOutMax=[]  FilterDiffOutCoefMin=[]  FilterDiffOutCoefMax=[]  ReciprocalOutMin=[]  ReciprocalOutMax=[]  SumDenOutMin=[]  SumDenOutMax=[]  SumNumOutMin=[]  SumNumOutMax=[]  DivideOutMin=[]  DivideOutMax=[]  UdiffTsProdOutMin=[]  UdiffTsProdOutMax=[]  NTsProdOutMin=[]  NTsProdOutMax=[]  UintegralTsProdOutMin=[]  UintegralTsProdOutMax=[]  UngainTsProdOutMin=[]  UngainTsProdOutMax=[]  IntegratorContinuousStateAttributes=''  IntegratorStateMustResolveToSignalObject=off  IntegratorRTWStateStorageClass=Auto  FilterContinuousStateAttributes=''  FilterStateMustResolveToSignalObject=off  FilterRTWStateStorageClass=Auto  ParallelPVariant=InternalParameters  IdealPVariant=Disabled  IVariant=InternalParameters  DVariant=Disabled  IntegratorVariant=Continuous  SatVariant=Disabled  AWVariant=Passthrough  PCopyVariant=Disabled  TRVariant=Disabled  FdbkBlocksVariant=Forward  IdealPFdbkVariant=Disabled  SatFdbkVariant=Disabled  DerivativeFilterVariant=Disabled  NVariant=Disabled  NCopyVariant=Disabled_SignalSpec  FilterICVariant=Disabled  IntegratorICVariant=InternalICs  ExternalResetVariant=Disabled  TRSumVariant=Passthrough  SumFdbkVariant=Disabled  SumVariant=Sum_PI  TsampFilterVariant=InternalTs  TsampNgainVariant=Passthrough  TsampIntegralVariant=Passthrough  ExternalSaturationOutDataTypeStr=Inherit: Same as second input
  Scope : Scope  NumInputPorts=3
  Vdq : Outport
  wires:
  Integrator2/1 -> Clarke to Park Angle Transform/2, Scope/3  "\\theta"
  Clarke Transform/1 -> Clarke to Park Angle Transform/1
  Clarke to Park Angle Transform/1 -> Scope/1, Demux1/1, Demux/1
  We/1 -> Add/2
  Demux/2 -> PID Controller/1  "Vq"
  PID Controller/1 -> Scope/2, Add/1  "W"
  Add/1 -> Integrator2/1  "W"
  Vabc/1 -> Clarke Transform/1
  Mux/1 -> Vdq/1
  Demux1/2 -> Mux/2
  Demux1/1 -> Mux/1

== system Inverter_circuit_redesign_from_NITW_Paper23_compatible/abd to dp Transform1 ==
  Iabc : Inport
  θe : Inport  Port=2
  Clarke Transform : eeTransforms/Clarke Transform  PowerInvariant=off
      settings: SourceProductBaseCode=PS
  Clarke to Park Angle Transform : eeTransforms/Clarke to Park Angle Transform  AxisAlignment=Q-axis
      settings: SourceProductBaseCode=PS
  Demux1 : Demux  Outputs=3
  Mux : Mux  Inputs=2
  Idq : Outport
  wires:
  Clarke Transform/1 -> Clarke to Park Angle Transform/1
  Clarke to Park Angle Transform/1 -> Demux1/1
  Iabc/1 -> Clarke Transform/1
  Demux1/2 -> Mux/2  "Iq"
  Demux1/1 -> Mux/1  "Id"
  θe/1 -> Clarke to Park Angle Transform/2
  Mux/1 -> Idq/1

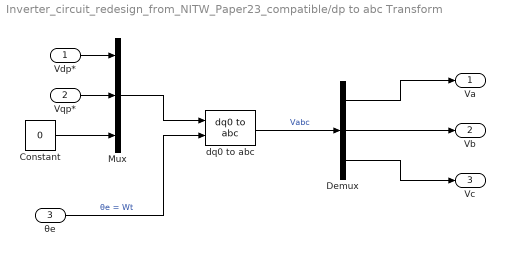
== system Inverter_circuit_redesign_from_NITW_Paper23_compatible/dp to abc Transform ==
  Vdp* : Inport
  Vqp* : Inport  Port=2
  θe : Inport  Port=3
  Constant : Constant  Value=0
  Demux : Demux  Outputs=3
  Mux : Mux  Inputs=3
  dq0 to abc : spsdq0toabcLib/dq0 to abc  Alignment=Aligned with phase A axis
  Va : Outport
  Vb : Outport  Port=2
  Vc : Outport  Port=3
  wires:
  Vqp*/1 -> Mux/2
  Vdp*/1 -> Mux/1
  Constant/1 -> Mux/3
  Mux/1 -> dq0 to abc/1
  dq0 to abc/1 -> Demux/1  "Vabc"
  θe/1 -> dq0 to abc/2  "θe = Wt"
  Demux/1 -> Va/1
  Demux/2 -> Vb/1
  Demux/3 -> Vc/1

== system Inverter_circuit_redesign_from_NITW_Paper23_compatible/LIM/Electromech Force ==
  note: Fe=(3*pi/2*t)*(P/2)*[ λdsIqs-λqsIds]
  λdqp : Inport
  Idqp : Inport  Port=2
  Add : Sum  Inputs=+-
  Constant2 : Constant  Value=3*pi*P/(4*Tp)
  Demux : Demux  Outputs=2
  Demux1 : Demux  Outputs=2
  Product : Product
  Product1 : Product
  Product2 : Product
  Fe : Outport
  wires:
  Product/1 -> Fe/1
  λdqp/1 -> Demux/1
  Idqp/1 -> Demux1/1
  Add/1 -> Product/2
  Demux/1 -> Product1/1  "λds"
  Demux1/2 -> Product1/2  "Iqs"
  Demux/2 -> Product2/1  "λqs"
  Demux1/1 -> Product2/2  "Ids"
  Product1/1 -> Add/1
  Product2/1 -> Add/2
  Constant2/1 -> Product/1

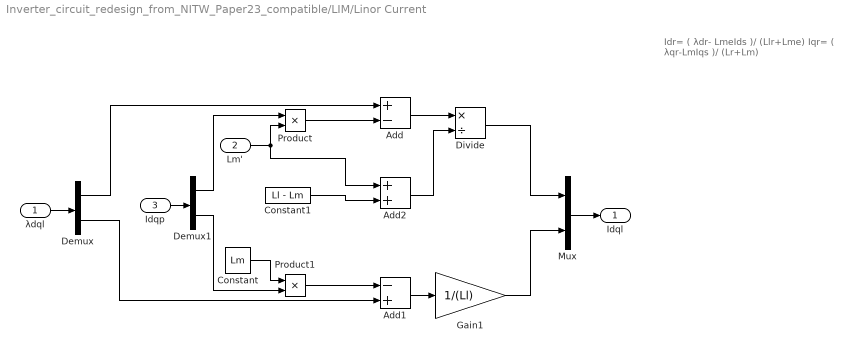
== system Inverter_circuit_redesign_from_NITW_Paper23_compatible/LIM/Linor Current ==
  note: Idr= ( λdr- LmeIds )/ (Llr+Lme)
      |
      | Iqr= ( λqr-LmIqs )/ (Lr+Lm)
  λdql : Inport
  Lm' : Inport  Port=2
  Idqp : Inport  Port=3
  Add : Sum  Inputs=+-
  Add1 : Sum  Inputs=-+
  Add2 : Sum
  Constant : Constant  Value=Lm  VectorParams1D=off
  Constant1 : Constant  Value=Ll - Lm
  Demux : Demux  Outputs=2
  Demux1 : Demux  Outputs=2
  Divide : Product  Inputs=*/
  Gain1 : Gain  Gain=1/(Ll)
  Mux : Mux  Inputs=2
  Product : Product
  Product1 : Product
  Idql : Outport
  wires:
  Mux/1 -> Idql/1
  λdql/1 -> Demux/1
  Idqp/1 -> Demux1/1
  Demux1/1 -> Product/1
  Demux1/2 -> Product1/2
  Demux/1 -> Add/1
  Demux/2 -> Add1/2
  Product/1 -> Add/2
  Product1/1 -> Add1/1
  Add/1 -> Divide/1
  Add1/1 -> Gain1/1
  Gain1/1 -> Mux/2
  Divide/1 -> Mux/1
  Constant/1 -> Product1/1
  Constant1/1 -> Add2/2
  Lm'/1 -> Add2/1, Product/2
  Add2/1 -> Divide/2

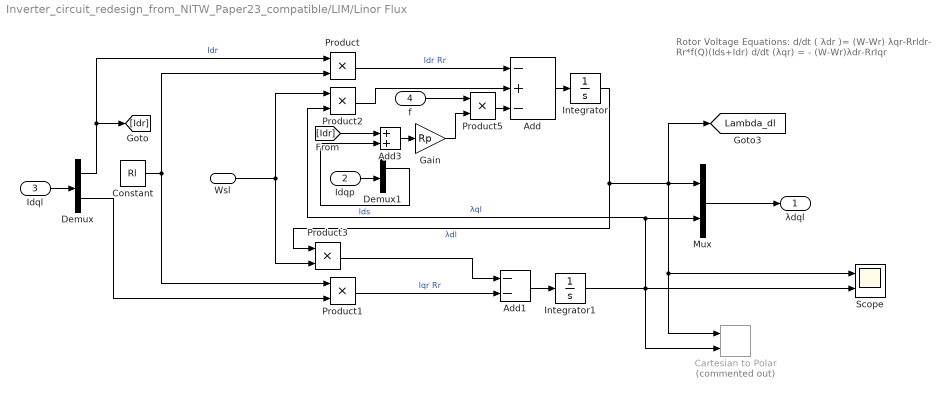
== system Inverter_circuit_redesign_from_NITW_Paper23_compatible/LIM/Linor Flux ==
  note: Rotor Voltage Equations:
      | d/dt ( λdr )= (W-Wr) λqr-RrIdr- Rr*f(Q)(Ids+Idr)
      | d/dt (λqr) = - (W-Wr)λdr-RrIqr
  Wsl : Inport
  Idqp : Inport  Port=2
  Idql : Inport  Port=3
  f : Inport  Port=4
  Add : Sum  Inputs=-+-
  Add1 : Sum  Inputs=--
  Add3 : Sum
  Cartesian to Polar : simulink_extras/Transformations/Cartesian to Polar  Commented=on
  Constant : Constant  Value=Rl
  Demux : Demux  Outputs=2
  Demux1 : Demux  Outputs=2
  Gain : Gain  Gain=Rp
  Integrator : Integrator
  Integrator1 : Integrator
  Mux : Mux  Inputs=2
  Product{,1..3,5} (5 alike) : Product
  Scope : Scope  NumInputPorts=2
  λdql : Outport
  tag scope: Lambda_dl=global
  wires:
  Mux/1 -> λdql/1
  Idql/1 -> Demux/1
  Demux/1 -> [Idr], Product/1  "Idr"
  Demux/2 -> Product1/2
  Constant/1 -> Product1/1, Product/2
  Product/1 -> Add/1  "Idr Rr"
  Product1/1 -> Add1/2  "Iqr Rr"
  Add/1 -> Integrator/1
  Add1/1 -> Integrator1/1
  Wsl/1 -> Product3/2, Product2/1
  Product2/1 -> Add/2
  Product3/1 -> Add1/1
  Demux1/1 -> Add3/2  "Ids"
  Product5/1 -> Add/3
  Add3/1 -> Gain/1
  Gain/1 -> Product5/2
  f/1 -> Product5/1
  Idqp/1 -> Demux1/1
  [Idr] -> Add3/1
  Integrator1/1 -> Product2/2, Mux/2, Scope/2, Cartesian to Polar/2  "λql"
  Integrator/1 -> Product3/1, [Lambda_dl], Cartesian to Polar/1, Scope/1, Mux/1  "λdl"

== system Inverter_circuit_redesign_from_NITW_Paper23_compatible/LIM/Mechanical System ==
  note: d/dt (v) = 1/M* [Fe-Fl-B*v]
  Fe : Inport
  F-load : Inport  Port=2
  Add : Sum  Inputs=+-
  Gain : Gain  Gain=pi/Tp
  Gain1 : Gain  Gain=1/(k*M)
  Gain2 : Gain  Gain=B*k
  Integrator : Integrator
  Subtract : Sum  Inputs=+-
  V : Outport
  Wl : Outport  Port=2
  wires:
  Fe/1 -> Subtract/1
  F-load/1 -> Subtract/2
  Gain/1 -> Wl/1
  Subtract/1 -> Add/1
  Gain1/1 -> Integrator/1
  Integrator/1 -> Gain/1, V/1, Gain2/1  "v"
  Add/1 -> Gain1/1
  Gain2/1 -> Add/2

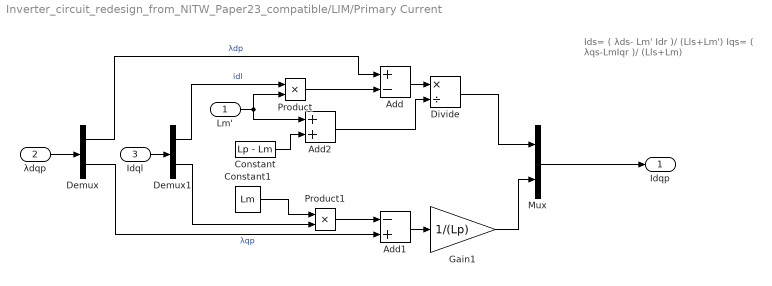
== system Inverter_circuit_redesign_from_NITW_Paper23_compatible/LIM/Primary Current ==
  note: Ids= ( λds- Lm' Idr )/ (Lls+Lm')
      |
      | Iqs= ( λqs-LmIqr )/ (Lls+Lm)
  Lm' : Inport
  λdqp : Inport  Port=2
  Idql : Inport  Port=3
  Add : Sum  Inputs=+-
  Add1 : Sum  Inputs=-+
  Add2 : Sum
  Constant : Constant  Value=Lp - Lm
  Constant1 : Constant  Value=Lm  VectorParams1D=off
  Demux : Demux  Outputs=2
  Demux1 : Demux  Outputs=2
  Divide : Product  Inputs=*/
  Gain1 : Gain  Gain=1/(Lp)
  Mux : Mux  Inputs=2
  Product : Product
  Product1 : Product
  Idqp : Outport
  wires:
  Demux/2 -> Add1/2  "λqp"
  Demux1/1 -> Product/1  "idl"
  Product/1 -> Add/2
  Product1/1 -> Add1/1
  λdqp/1 -> Demux/1
  Add1/1 -> Gain1/1
  Idql/1 -> Demux1/1
  Demux/1 -> Add/1  "λdp"
  Demux1/2 -> Product1/2
  Add/1 -> Divide/1
  Divide/1 -> Mux/1
  Gain1/1 -> Mux/2
  Constant1/1 -> Product1/1
  Lm'/1 -> Add2/1, Product/2
  Constant/1 -> Add2/2
  Add2/1 -> Divide/2
  Mux/1 -> Idqp/1

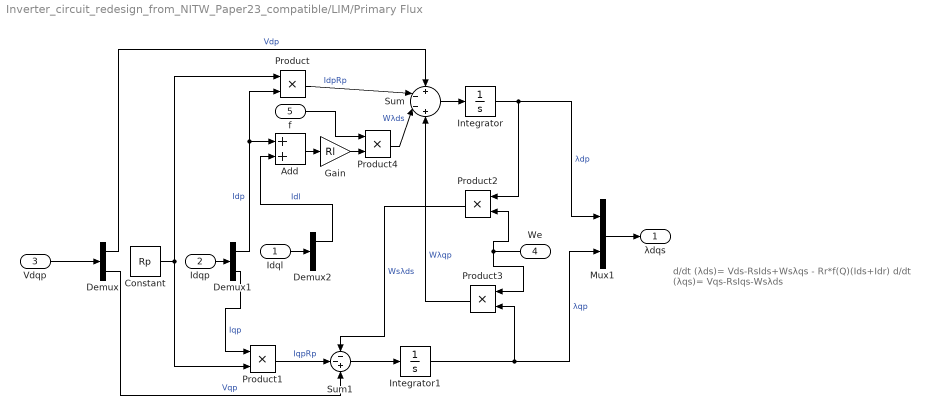
== system Inverter_circuit_redesign_from_NITW_Paper23_compatible/LIM/Primary Flux ==
  note: d/dt (λds)= Vds-RsIds+Wsλqs - Rr*f(Q)(Ids+Idr)
      |
      | d/dt (λqs)= Vqs-RsIqs-Wsλds
  Idql : Inport
  Idqp : Inport  Port=2
  Vdqp : Inport  Port=3
  We : Inport  Port=4
  f : Inport  Port=5
  Add : Sum
  Constant : Constant  Value=Rp
  Demux : Demux  Outputs=2
  Demux1 : Demux  Outputs=2
  Demux2 : Demux  Outputs=2
  Gain : Gain  Gain=Rl
  Integrator : Integrator
  Integrator1 : Integrator
  Mux1 : Mux  Inputs=2
  Product{,1..4} (5 alike) : Product
  Sum : Sum  Inputs=+--+
  Sum1 : Sum  Inputs=--+
  λdqs : Outport
  wires:
  Integrator1/1 -> Product3/2, Mux1/2  "λqp"
  Integrator/1 -> Product2/1, Mux1/1  "λdp"
  Vdqp/1 -> Demux/1
  Idqp/1 -> Demux1/1
  Demux/1 -> Sum/1  "Vdp"
  Sum/1 -> Integrator/1
  Constant/1 -> Product1/2, Product/1
  Demux1/1 -> Product/2, Add/1  "Idp"
  Product/1 -> Sum/2  "IdpRp"
  Sum1/1 -> Integrator1/1
  Demux/2 -> Sum1/3  "Vqp"
  Demux1/2 -> Product1/1  "Iqp"
  Product1/1 -> Sum1/2  "IqpRp"
  We/1 -> Product3/1, Product2/2
  Product3/1 -> Sum/4  "Wλqp"
  Product2/1 -> Sum1/1  "Wsλds"
  Mux1/1 -> λdqs/1
  Idql/1 -> Demux2/1
  Demux2/1 -> Add/2  "Idl"
  Add/1 -> Gain/1
  Gain/1 -> Product4/2
  Product4/1 -> Sum/3  "Wλds"
  f/1 -> Product4/1

== system Inverter_circuit_redesign_from_NITW_Paper23_compatible/LIM/Vabc to Vdq OLD  ==
  note: Vα=2/3*[Va-0.5*{Vb+Vc}]
      |
      | Vβ=2/3*[√3/2 *{Vb-Vc}]
  note: Vd= Vα*cos ρ + Vβ*sin ρ
      |
      | Vq= Vβ*cos ρ - Vα*sin ρ
  Vabc : Inport
  We : Inport  Port=2
  Demux : Demux  Outputs=3
  Integrator : Integrator
  MATLAB Function : MATLAB Function  TreatAsAtomicUnit=on
  Mux : Mux  Inputs=2
  Vdqs : Outport
  wires:
  Vabc/1 -> Demux/1
  Demux/1 -> MATLAB Function/1(Va)
  Demux/2 -> MATLAB Function/2(Vb)
  Demux/3 -> MATLAB Function/3(Vc)
  We/1 -> Integrator/1
  Integrator/1 -> MATLAB Function/4(Wt)  "Wt"
  Mux/1 -> Vdqs/1
  MATLAB Function/1(Vd) -> Mux/1
  MATLAB Function/2(Vq) -> Mux/2

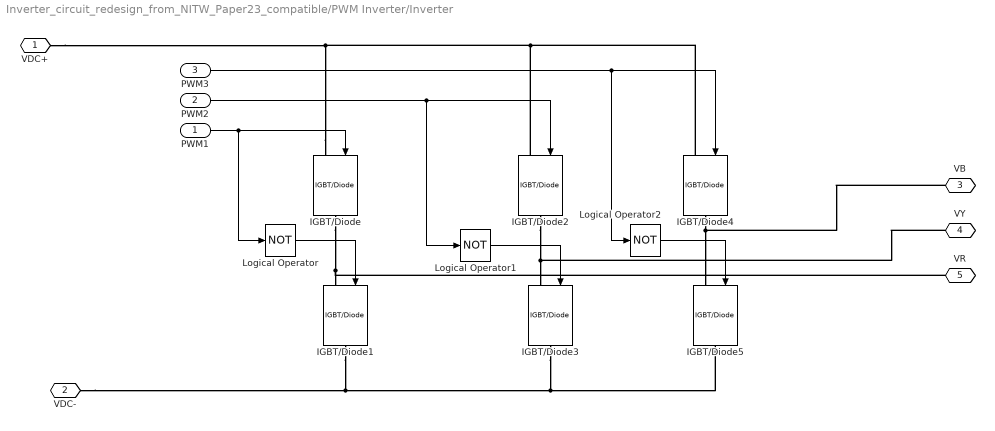
== system Inverter_circuit_redesign_from_NITW_Paper23_compatible/PWM Inverter/Inverter ==
  PWM1 : Inport
  PWM2 : Inport  Port=2
  PWM3 : Inport  Port=3
  IGBT/Diode{,1..5} (6 alike) : spsIGBTDiodeLib/IGBT//Diode  Ron=1e-3  Rs=1e5  Cs=inf  Measurements=off
  Logical Operator : Logic  Operator=NOT  AllPortsSameDT=off  OutDataTypeStr=boolean
  Logical Operator1 : Logic  Operator=NOT  AllPortsSameDT=off  OutDataTypeStr=boolean
  Logical Operator2 : Logic  Operator=NOT  AllPortsSameDT=off  OutDataTypeStr=boolean
  VDC+ : PMIOPort  Side=Left
  VDC- : PMIOPort  Port=2  Side=Left
  VB : PMIOPort  Port=3  Side=Right
  VY : PMIOPort  Port=4  Side=Right
  VR : PMIOPort  Port=5  Side=Right
  wires:
  PWM2/1 -> IGBT/Diode2/1, Logical Operator1/1
  Logical Operator/1 -> IGBT/Diode1/1
  PWM1/1 -> IGBT/Diode/1, Logical Operator/1
  PWM3/1 -> Logical Operator2/1, IGBT/Diode4/1
  Logical Operator2/1 -> IGBT/Diode5/1
  Logical Operator1/1 -> IGBT/Diode3/1
  connections:
  IGBT/Diode5/RConn1 -- VDC-/RConn1 -- IGBT/Diode1/RConn1 -- IGBT/Diode3/RConn1
  IGBT/Diode/LConn1 -- VDC+/RConn1 -- IGBT/Diode2/LConn1 -- IGBT/Diode4/LConn1
  IGBT/Diode/RConn1 -- VR/RConn1 -- IGBT/Diode1/LConn1
  IGBT/Diode2/RConn1 -- IGBT/Diode3/LConn1 -- VY/RConn1
  IGBT/Diode4/RConn1 -- IGBT/Diode5/LConn1 -- VB/RConn1

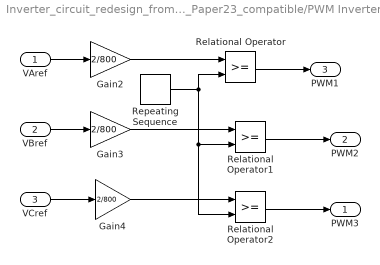
== system Inverter_circuit_redesign_from_NITW_Paper23_compatible/PWM Inverter/PMW ==
  VAref : Inport
  VBref : Inport  Port=2
  VCref : Inport  Port=3
  Gain2 : Gain  Gain=2/800
  Gain3 : Gain  Gain=2/800
  Gain4 : Gain  Gain=2/800
  Relational Operator : RelationalOperator  OutDataTypeStr=boolean  RndMeth=Simplest
  Relational Operator1 : RelationalOperator  OutDataTypeStr=boolean  RndMeth=Simplest
  Relational Operator2 : RelationalOperator  OutDataTypeStr=boolean  RndMeth=Simplest
  Repeating Sequence : simulink/Sources/Repeating Sequence  rep_seq_t=[0 0.00005 0.0001]  rep_seq_y=[-1 1 -1]
  PWM3 : Outport
  PWM2 : Outport  Port=2
  PWM1 : Outport  Port=3
  wires:
  Relational Operator1/1 -> PWM2/1
  Gain2/1 -> Relational Operator/1
  Gain4/1 -> Relational Operator2/1
  VAref/1 -> Gain2/1
  Relational Operator2/1 -> PWM3/1
  Repeating Sequence/1 -> Relational Operator2/2, Relational Operator1/2, Relational Operator/2
  Gain3/1 -> Relational Operator1/1
  VCref/1 -> Gain4/1
  VBref/1 -> Gain3/1
  Relational Operator/1 -> PWM1/1

== matlab function Inverter_circuit_redesign_from_NITW_Paper23_compatible/LIM/Vabc to Vdq OLD /MATLAB Function ==
  data: Va input; Vd output; Vb input; Vc input; Wt input; Vq output
function [Vd,Vq] = Transform(Va, Vb, Vc, Wt)
    M = [cos(Wt)    cos(Wt - 2*pi/3)    cos(Wt-4*pi/3);
        -sin(Wt)    -sin(Wt- 2*pi/3)    -sin(Wt-4*pi/3);
        1/sqrt(2)       1/sqrt(2)           1/sqrt(2)];
    
    DQ = M*[Va,Vb,Vc]';
    
    Vd = DQ(1);
    Vq = DQ(2);
end

== matlab function Inverter_circuit_redesign_from_NITW_Paper23_compatible/LIM/MATLAB Function ==
  data: v input; Lme output; Rl input; D input; Ll input; Lm input; f output
function [Lme,f]= fcn(v, Rl,D,Ll,Lm)
Q=abs((D*Rl)/(Ll*v));

f=(1-(exp(-Q)))/Q;

Lme = Lm*(1-f);

== matlab function Inverter_circuit_redesign_from_NITW_Paper23_compatible/LIM/MATLAB Function1 ==
  data: Iqp_star input; vsl output; Idp_star input; f input; Tp input; Ll input; Rl input; Lm input
function vsl = vsl_calculation(Iqp_star, Idp_star, f, Tp, Ll, Rl, Lm)
    
    vsl = Tp*(1 - f)*Iqp_star/(pi*(Ll/Rl - Lm*f/Rl)*Idp_star);

end
